simulink model "CubeSat_RWA_Simple"  (R2024b)
settings: Solver=ode4  StartTime=0.0  StopTime=100  FixedStep=T_sample  RelTol=1e-3
values from neighbouring files (symbols this model uses):
  Init_Quat = [1; 0; 0; 0]    [init_sim.m]
  Init_Rates = [0.0; -n_orbit; 0.0]    [init_sim.m]
  Init_Wheel_Speed = [0; 0; 0]    [init_sim.m]
  J_body = diag([0.002, 0.002, 0.002])    [init_sim.m]
  J_inv = inv(J_body)    [init_sim.m]
  J_wheel = diag([J_w_val, J_w_val, J_w_val])    [init_sim.m]
  J_wheel_inv = inv(J_wheel)    [init_sim.m]
  Kd = 8e-3    (= 0.008)    [init_sim.m]
  Kp = 5e-4    (= 0.0005)    [init_sim.m]
  Tau_Max = 1e-3    (= 0.001)    [init_sim.m]
settings Model: Creator=abdel  LastModifiedBy=abdel

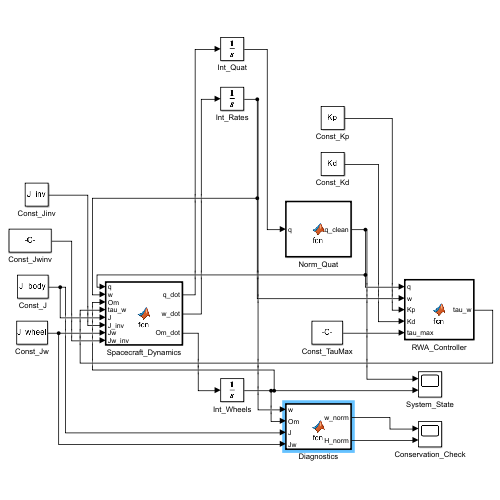
[thumbnail: Simulink's stored preview of the top-level diagram]
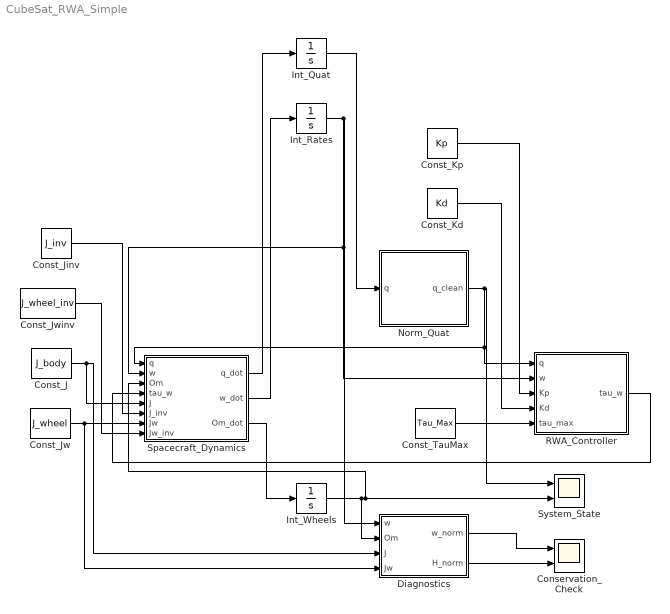
== system CubeSat_RWA_Simple ==
  Conservation_Check : Scope  NumInputPorts=2
  Const_J : Constant  Value=J_body
  Const_Jinv : Constant  Value=J_inv
  Const_Jw : Constant  Value=J_wheel
  Const_Jwinv : Constant  Value=J_wheel_inv
  Const_Kd : Constant  Value=Kd
  Const_Kp : Constant  Value=Kp
  Const_TauMax : Constant  Value=Tau_Max
  Diagnostics : MATLAB Function  TreatAsAtomicUnit=on
  Int_Quat : Integrator  InitialCondition=Init_Quat
  Int_Rates : Integrator  InitialCondition=Init_Rates
  Int_Wheels : Integrator  InitialCondition=Init_Wheel_Speed
  Norm_Quat : MATLAB Function  TreatAsAtomicUnit=on
  RWA_Controller : MATLAB Function  TreatAsAtomicUnit=on
  Spacecraft_Dynamics : MATLAB Function  TreatAsAtomicUnit=on
  System_State : Scope  NumInputPorts=2
  wires:
  Const_Jinv/1 -> Spacecraft_Dynamics/6(J_inv)
  Int_Quat/1 -> Norm_Quat/1(q)
  Const_Jwinv/1 -> Spacecraft_Dynamics/8(Jw_inv)
  Spacecraft_Dynamics/3(Om_dot) -> Int_Wheels/1
  Const_J/1 -> Diagnostics/3(J), Spacecraft_Dynamics/5(J)
  Const_Kd/1 -> RWA_Controller/4(Kd)
  Const_Jw/1 -> Diagnostics/4(Jw), Spacecraft_Dynamics/7(Jw)
  Spacecraft_Dynamics/2(w_dot) -> Int_Rates/1
  Spacecraft_Dynamics/1(q_dot) -> Int_Quat/1
  Int_Rates/1 -> RWA_Controller/2(w), Spacecraft_Dynamics/2(w), Diagnostics/1(w)
  Int_Wheels/1 -> Spacecraft_Dynamics/3(Om), System_State/2, Diagnostics/2(Om)
  Const_Kp/1 -> RWA_Controller/3(Kp)
  Norm_Quat/1(q_clean) -> Spacecraft_Dynamics/1(q), RWA_Controller/1(q), System_State/1
  Const_TauMax/1 -> RWA_Controller/5(tau_max)
  Diagnostics/1(w_norm) -> Conservation_Check/1
  Diagnostics/2(H_norm) -> Conservation_Check/2
  RWA_Controller/1(tau_w) -> Spacecraft_Dynamics/4(tau_w)

== matlab function CubeSat_RWA_Simple/Spacecraft_Dynamics ==
  data: q input; q_dot output; w input; Om input; tau_w input; J input; J_inv input; Jw input; Jw_inv input; w_dot output; Om_dot output
function [q_dot, w_dot, Om_dot] = fcn(q, w, Om, tau_w, J, J_inv, Jw, Jw_inv)
    q = q(:); w = w(:); Om = Om(:); tau_w = tau_w(:);
    
    % Kinematics
    q_dot = 0.5 * [ -q(2)*w(1) - q(3)*w(2) - q(4)*w(3);
                     q(1)*w(1) - q(4)*w(2) + q(3)*w(3);
                     q(4)*w(1) + q(1)*w(2) - q(2)*w(3);
                    -q(3)*w(1) + q(2)*w(2) + q(1)*w(3) ];
    
    % Dynamics
    H = J*w + Jw*Om;
    w_dot = J_inv * ( -tau_w - cross(w, H) );
    Om_dot = Jw_inv * tau_w;
end

== matlab function CubeSat_RWA_Simple/RWA_Controller ==
  data: q input; tau_w output; w input; Kp input; Kd input; tau_max input
function tau_w = fcn(q, w, Kp, Kd, tau_max)
    % Define output immediately to prevent errors
    tau_w = zeros(3,1);
    q = q(:); w = w(:);
    
    % Error calc
    qe = q;
    if qe(1) < 0
        qe = -qe;
    end
    
    % PD Control
    e_vec = qe(2:4);
    tau_body_cmd = -Kp * e_vec - Kd * w;
    tau_w_raw = -tau_body_cmd;
    
    % Saturation
    for i=1:3
        tau_w(i) = max(min(tau_w_raw(i), tau_max), -tau_max);
    end
end

== matlab function CubeSat_RWA_Simple/Norm_Quat ==
  data: q input; q_clean output
function q_clean = fcn(q)
    q = q(:);
    n = norm(q);
    if n < 1e-12, n = 1; end
    q_clean = q / n;
end

== matlab function CubeSat_RWA_Simple/Diagnostics ==
  data: w input; w_norm output; Om input; J input; Jw input; H_norm output
function [w_norm, H_norm] = fcn(w, Om, J, Jw)
    w = w(:); Om = Om(:);
    H = J*w + Jw*Om;
    w_norm = norm(w);
    H_norm = norm(H);
end
